simulink model "JCBL_Buck_Verify"  (R2024b)
settings: Solver=VariableStepAuto  StartTime=0.0  StopTime=0.5  RelTol=1e-3
undefined symbols (not defined in the file): C, L, RC, RL
libraries: spsCurrentMeasurementLib x9, spsMeanLib x6, spsVoltageMeasurementLib x6, spsSeriesRLCBranchLib x5, spsMosfetLib x4, spsOnDelayLib x4, slpidlib x3, simulink x3, eePowerMeasurement x2, spsRMSLib x2, spsControlledVoltageSourceLib x1, spsDCVoltageSourceLib x1
settings Model: Creator=admin  LastModifiedBy=admin
settings SolverCC: ZeroCrossAlgorithm=Adaptive  AlgebraicLoopSolver=TrustRegion
settings DebuggingCC: UnconnectedInputMsg=warning  UnconnectedOutputMsg=warning  UnconnectedLineMsg=warning
settings ModelReferenceCC: EnableRefExpFcnMdlSchedulingChecks=on
settings RTWCC: GPUComputeCapability=3.5  DLArmComputeVersion=19.05

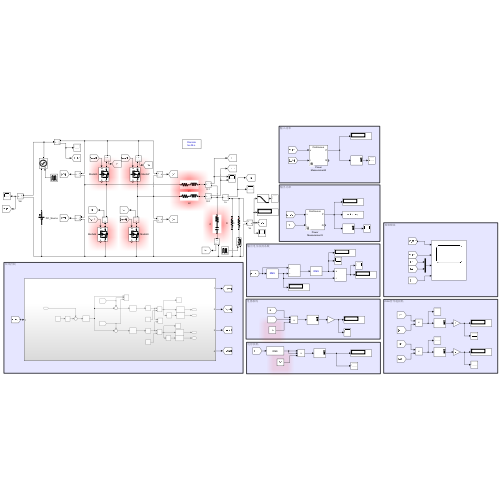
[thumbnail: Simulink's stored preview of the top-level diagram]
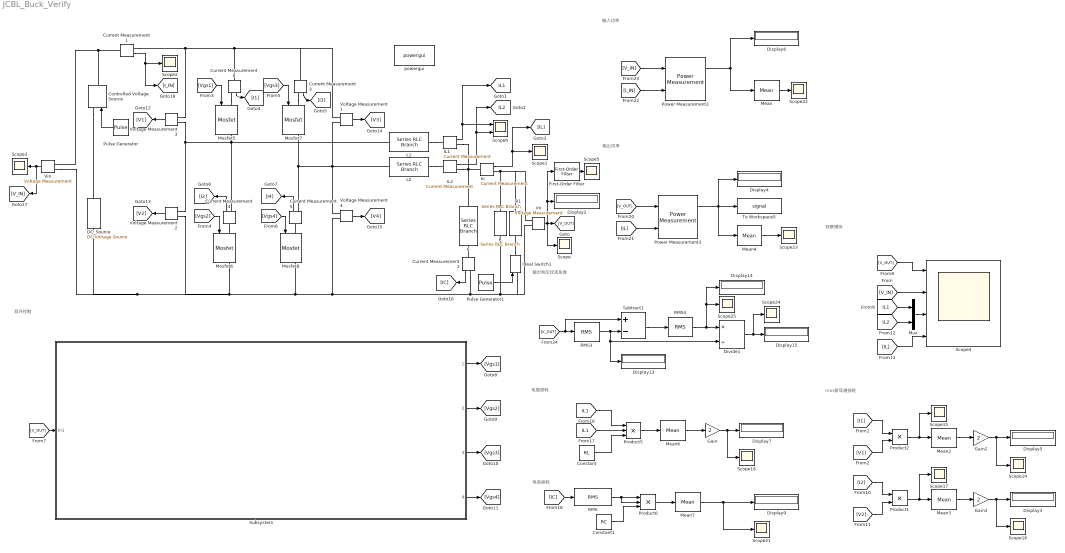
== system JCBL_Buck_Verify ==
  note: mos管导通损耗
  note: 电容损耗
  note: 电感损耗
  note: 输入功率
  note: 输出电压纹波系数
  note: 双环控制
  note: 输出功率
  note: 观察模块
  C : spsSeriesRLCBranchLib/Series RLC Branch  LConnTagsString=__new0  RConnTagsString=__new0  BranchType=RC  Resistance=RC  Inductance=1e-3  SetiL0=off  InitialCurrent=0  Capacitance=C  Setx0=off  InitialVoltage=0  Measurements=None
  Constant : Constant  Value=RL
  Constant1 : Constant  Value=RC
  Controlled Voltage Source : spsControlledVoltageSourceLib/Controlled Voltage Source  Initialize=on  Source_Type=AC  Amplitude=0  Phase=0  Frequency=0  Measurements=None
  Current Measurement{1..6} (6 alike) : spsCurrentMeasurementLib/Current Measurement  PhasorSimulation=off  OutputType=Complex  PSBequivalent=0
  DC_Source : spsDCVoltageSourceLib/DC Voltage Source  Amplitude=48  Measurements=None
  Display{2..7,9,13..15} (10 alike) : Display
  Divide1 : Product  Inputs=*/
  First-Order Filter : spsFirstOrderFilterLib/First-Order Filter  FilterType=Lowpass  Tc=1.26e-5  Ts=0  Initialize=off  Vac_Init=[0, 0, 60]  Vdc_Init=0  PlotResponse=off  FreqRange="[0,  200,  1]"
  Gain : Gain  Gain=2
  Gain2 : Gain  Gain=2
  Gain3 : Gain  Gain=2
  IL1 : spsCurrentMeasurementLib/Current Measurement  PhasorSimulation=off  OutputType=Complex  PSBequivalent=0
  IL2 : spsCurrentMeasurementLib/Current Measurement  PhasorSimulation=off  OutputType=Complex  PSBequivalent=0
  Ideal Switch1 : spsIdealSwitchLib/Ideal Switch  Ron=0.001  Lon=0  IC=0  Rs=1e5  Cs=inf  Measurements=off
  Io : spsCurrentMeasurementLib/Current Measurement  PhasorSimulation=off  OutputType=Complex  PSBequivalent=0
  L1 : spsSeriesRLCBranchLib/Series RLC Branch  LConnTagsString=__new0  RConnTagsString=__new0  BranchType=RL  Resistance=RL  Inductance=L  SetiL0=off  InitialCurrent=0  Capacitance=1e-6  Setx0=off  InitialVoltage=0  Measurements=None
  L2 : spsSeriesRLCBranchLib/Series RLC Branch  LConnTagsString=__new0  RConnTagsString=__new0  BranchType=RL  Resistance=RL  Inductance=L  SetiL0=off  InitialCurrent=0  Capacitance=1e-6  Setx0=off  InitialVoltage=0  Measurements=None
  Mean{,2..4,6..7} (6 alike) : spsMeanLib/Mean  Freq=500000  Vinit=0  Ts=0
  Mosfet{5..8} (4 alike) : spsMosfetLib/Mosfet  Ron=Ron  Lon=0  Rd=0.0001  Vfd=0  IC=0  Rs=1e5  Cs=inf  Measurements=on
  Mux : Mux  Inputs=2
  Power Measurement2 : eePowerMeasurement/Power Measurement  LabelModeActiveChoice=Continuous  F=60  K=[0]  Ts=0
  Power Measurement3 : eePowerMeasurement/Power Measurement  LabelModeActiveChoice=Continuous  F=60  K=[0]  Ts=0
  Product1 : Product
  Product2 : Product
  Product5 : Product  Inputs=3
  Product6 : Product  Inputs=3
  Pulse Generator : DiscretePulseGenerator  PulseType=Time based  Amplitude=4  Period=1  PulseWidth=15  PhaseDelay=0.25
  Pulse Generator1 : DiscretePulseGenerator  PulseType=Time based  Amplitude=4  Period=0.18  PulseWidth=1/3*100  PhaseDelay=0.16
  R : spsSeriesRLCBranchLib/Series RLC Branch  LConnTagsString=__new0  RConnTagsString=__new0  BranchType=R  Resistance=0.14  Inductance=1e-3  SetiL0=off  InitialCurrent=0  Capacitance=1e-6  Setx0=off  InitialVoltage=0  Measurements=None
  R1 : spsSeriesRLCBranchLib/Series RLC Branch  LConnTagsString=__new0  RConnTagsString=__new0  BranchType=R  Resistance=0.14  Inductance=1e-3  SetiL0=off  InitialCurrent=0  Capacitance=1e-6  Setx0=off  InitialVoltage=0  Measurements=None
  RMS : dspstat3/RMS  run=off  directionMode=Each column  dimension=1  InputProcessing=Columns as channels (frame based)  reset_popup=None
  RMS3 : spsRMSLib/RMS  TrueRMS=on  Freq=60  RMSInit=0  Ts=0
  RMS4 : spsRMSLib/RMS  TrueRMS=on  Freq=60  RMSInit=0  Ts=0
  Scope{,1..3,5,14..18,21..25} (15 alike) : Scope
  Scope4 : Scope  NumInputPorts=4
  Scope6 : Scope  NumInputPorts=2
  Subsystem : Subsystem
  Subtract1 : Sum  Inputs=+-
  To Workspace5 : ToWorkspace  VariableName=signal  SampleTime=0.1
  Vin : spsVoltageMeasurementLib/Voltage Measurement  PhasorSimulation=off  OutputType=Complex  PSBequivalent=0
  Vo : spsVoltageMeasurementLib/Voltage Measurement  PhasorSimulation=off  OutputType=Complex  PSBequivalent=0
  Voltage Measurement{1..4} (4 alike) : spsVoltageMeasurementLib/Voltage Measurement  PhasorSimulation=off  OutputType=Complex  PSBequivalent=0
  powergui : spspowerguiLib/powergui  Priority=1  SimulationMode=Discrete  SampleTime=5e-8  frequency=60  Iterations=50  frequencyindice=0  Pbase=100e6  ErrMax=1e-4  UnitsV=kV  UnitsW=MW  buscounter=0  FunctionMessages=off  echomessages=off  EnableUseOfTLC=off  CurrentSourceSwitches=off  DisableSnubberDevices=off  DisableRonSwitches=off  DisableVfSwitches=off  DisplayEquations=off  AutomaticDiscreteSolvers=off  SolverType=Tustin/Backward Euler (TBE)  Interpol=off  ExternalGateDelay=off  methode=off  Ts=100  x0status=blocks  SPID=on  SwTol=0  HookPort=off  NonlinearTolerance=1e-4  nMaxIteration=100  ContinueOnMaxIteration=off  RestoreLinks=warning  ResistiveCurrentMeasurement=off  Frange=[0:2:500]  Ylog=off  Xlog=on  ShowGrid=off  save=off  variable=ZData  structure=0  ZoomFFT=off  StartTime=0.0  cycles=1  DisplayStyle=1  fundamental=60  FreqAxis=off  MaxFrequency=1000  frequencyindicesteady=1  RmsSteady=1  display=off
  tag scope: IL1=global, IL2=global
  wires:
  Pulse Generator/1 -> Controlled Voltage Source/1
  Pulse Generator1/1 -> Ideal Switch1/1
  Gain3/1 -> Display3/1, Scope16/1
  Mean3/1 -> Gain3/1
  Gain2/1 -> Display5/1, Scope14/1
  Mean2/1 -> Gain2/1
  [I2] -> Product1/1
  [V2] -> Product1/2
  Product1/1 -> Mean3/1, Scope17/1
  Product2/1 -> Scope15/1, Mean2/1
  [V1] -> Product2/2
  [I1] -> Product2/1
  RMS/1 -> Product6/1, Product6/2
  Mean7/1 -> Display9/1, Scope21/1
  Product6/1 -> Mean7/1
  Constant1/1 -> Product6/3
  [IC] -> RMS/1
  Gain/1 -> Display7/1, Scope18/1
  Mean6/1 -> Gain/1
  Product5/1 -> Mean6/1
  Constant/1 -> Product5/3
  [IL1] -> Product5/2
  [IL1] -> Product5/1
  [V_IN] -> Power Measurement2/1
  [I_IN] -> Power Measurement2/2
  [IL] -> Power Measurement3/2
  [V_OUT] -> Power Measurement3/1
  Mean4/1 -> Scope23/1
  Power Measurement3/1 -> To Workspace5/1, Display4/1, Mean4/1
  Power Measurement2/1 -> Mean/1, Display6/1
  Mean/1 -> Scope22/1
  [V_OUT] -> Subtract1/1, RMS3/1
  RMS3/1 -> Subtract1/2, Divide1/2, Display13/1
  Subtract1/1 -> RMS4/1
  RMS4/1 -> Divide1/1, Display14/1, Scope25/1
  Divide1/1 -> Scope24/1, Display15/1
  [V_OUT] -> Subsystem/1(In1)
  Subsystem/4(4) -> [Vgs4]
  Subsystem/1(1) -> [Vgs1]
  Subsystem/2(2) -> [Vgs2]
  Subsystem/3(3) -> [Vgs3]
  [Vgs1] -> Mosfet5/1
  [Vgs3] -> Mosfet7/1
  Current Measurement5/1 -> [I4]
  Current Measurement6/1 -> [I1]
  Voltage Measurement4/1 -> [V4]
  Voltage Measurement3/1 -> [V1]
  [Vgs2] -> Mosfet6/1
  Voltage Measurement1/1 -> [V3]
  Voltage Measurement2/1 -> [V2]
  Current Measurement3/1 -> [I3]
  [Vgs4] -> Mosfet8/1
  Current Measurement4/1 -> [I2]
  Current Measurement2/1 -> [IC]
  Vin/1 -> [V_IN], Scope3/1
  Current Measurement1/1 -> Scope2/1, [I_IN]
  IL1/1 -> [IL1], Scope6/1
  IL2/1 -> [IL2], Scope6/2
  Io/1 -> [IL], Scope1/1
  Vo/1 -> Scope/1, First-Order Filter/1, Display2/1, [V_OUT]
  [IL1] -> Mux/1
  [IL2] -> Mux/2
  [V_OUT] -> Scope4/1
  [V_IN] -> Scope4/2
  Mux/1 -> Scope4/3
  [IL] -> Scope4/4
  First-Order Filter/1 -> Scope5/1
  connections:
  Current Measurement2/RConn1 -- Voltage Measurement4/LConn1 -- Voltage Measurement2/LConn1 -- Vin/LConn2 -- DC_Source/LConn1 -- Mosfet6/RConn1 -- Mosfet8/RConn1 -- Ideal Switch1/LConn1 -- Vo/LConn2 -- R/RConn1
  Controlled Voltage Source/RConn1 -- Vin/LConn1 -- Current Measurement1/LConn1
  C/LConn1 -- IL1/RConn1 -- Io/LConn1 -- IL2/RConn1
  Io/RConn1 -- R1/LConn1 -- Vo/LConn1 -- R/LConn1
  L2/RConn1 -- IL2/LConn1
  L1/RConn1 -- IL1/LConn1
  Current Measurement2/LConn1 -- C/RConn1
  Controlled Voltage Source/LConn1 -- DC_Source/RConn1
  Voltage Measurement3/LConn2 -- Voltage Measurement2/LConn2 -- L1/LConn1 -- Mosfet5/RConn1 -- Current Measurement4/RConn1
  Voltage Measurement1/LConn2 -- Voltage Measurement4/LConn2 -- Current Measurement5/RConn1 -- Mosfet7/RConn1 -- L2/LConn1
  Current Measurement4/LConn1 -- Mosfet6/LConn1
  Mosfet8/LConn1 -- Current Measurement5/LConn1
  Current Measurement3/RConn1 -- Mosfet7/LConn1
  Current Measurement6/RConn1 -- Mosfet5/LConn1
  Current Measurement1/RConn1 -- Voltage Measurement3/LConn1 -- Current Measurement3/LConn1 -- Voltage Measurement1/LConn1 -- Current Measurement6/LConn1
  Ideal Switch1/RConn1 -- R1/RConn1

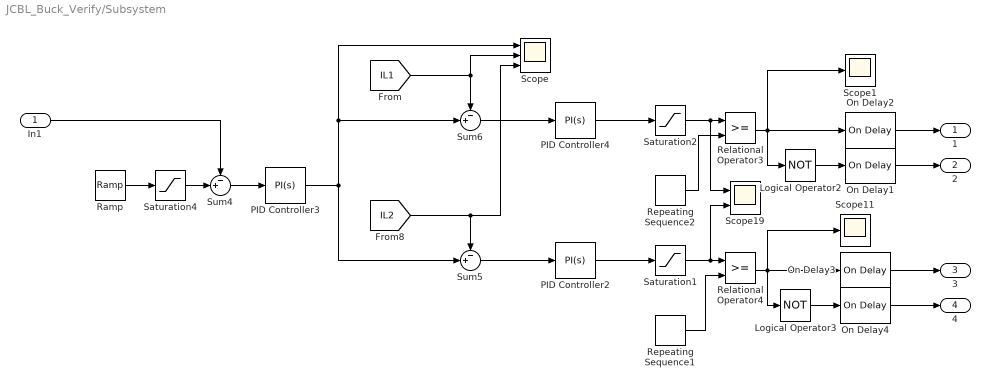
== system JCBL_Buck_Verify/Subsystem ==
  In1 : Inport
  Logical Operator2 : Logic  Operator=NOT  AllPortsSameDT=off  OutDataTypeStr=boolean
  Logical Operator3 : Logic  Operator=NOT  AllPortsSameDT=off  OutDataTypeStr=boolean
  On Delay{1..4} (4 alike) : spsOnDelayLib/On Delay  DelayType=On delay  delay=100e-9  ic=0  Ts=0
  PID Controller2 : slpidlib/PID Controller  Controller=PI  Form=Parallel  TimeDomain=Continuous-time  UseExternalTs=off  SampleTime=-1  IntegratorMethod=Forward Euler  FilterMethod=Forward Euler  ControllerParametersSource=internal  P=0.2  I=8  UseKiTs=off  D=0  UseExternalDerivativeSource=off  N=100  UseFilter=on  TunerSelectOption=Transfer Function Based (PID Tuner App)  InitialConditionSource=internal  InitialConditionForIntegrator=0  InitialConditionForFilter=0  DifferentiatorICPrevScaledInput=0  ExternalReset=none  TrackingMode=off  Kt=1  LimitOutput=on  SatLimitsSource=internal  UpperSaturationLimit=0.98  LowerSaturationLimit=0  LinearizeAsGain=on  AntiWindupMode=none  Kb=1  LimitIntegrator=off  UpperIntegratorSaturationLimit=0.95  LowerIntegratorSaturationLimit=0.05  POutMin=[]  POutMax=[]  IOutMin=[]  IOutMax=[]  DOutMin=[]  DOutMax=[]  NOutMin=[]  NOutMax=[]  SumOutMin=[]  SumOutMax=[]  SaturationOutMin=[]  SaturationOutMax=[]  PParamMin=[]  PParamMax=[]  IParamMin=[]  IParamMax=[]  DParamMin=[]  DParamMax=[]  NParamMin=[]  NParamMax=[]  KbParamMin=[]  KbParamMax=[]  KtParamMin=[]  KtParamMax=[]  KbOutMin=[]  KbOutMax=[]  KtOutMin=[]  KtOutMax=[]  IntegratorOutMin=[]  IntegratorOutMax=[]  FilterOutMin=[]  FilterOutMax=[]  SumI1OutMin=[]  SumI1OutMax=[]  SumI2OutMin=[]  SumI2OutMax=[]  SumI3OutMin=[]  SumI3OutMax=[]  SumI4OutMin=[]  SumI4OutMax=[]  SumDOutMin=[]  SumDOutMax=[]  DifferentiatorOutMin=[]  DifferentiatorOutMax=[]  FilterDiffOutCoefMin=[]  FilterDiffOutCoefMax=[]  ReciprocalOutMin=[]  ReciprocalOutMax=[]  SumDenOutMin=[]  SumDenOutMax=[]  SumNumOutMin=[]  SumNumOutMax=[]  DivideOutMin=[]  DivideOutMax=[]  UdiffTsProdOutMin=[]  UdiffTsProdOutMax=[]  NTsProdOutMin=[]  NTsProdOutMax=[]  UintegralTsProdOutMin=[]  UintegralTsProdOutMax=[]  UngainTsProdOutMin=[]  UngainTsProdOutMax=[]  ClampingZeroOutDataTypeStr=Inherit: Inherit via back propagation  ClampingZeroOutMin=[]  ClampingZeroOutMax=[]  FilterDenConstantOutDataTypeStr=Inherit: Inherit via back propagation  FilterDenConstantOutMin=[]  FilterDenConstantOutMax=[]  PCopyOutDataTypeStr=Inherit: Inherit via back propagation  PCopyOutMin=[]  PCopyOutMax=[]  NCopyOutDataTypeStr=Inherit: Inherit via back propagation  NCopyOutMin=[]  NCopyOutMax=[]  IntegratorContinuousStateAttributes=''  IntegratorStateMustResolveToSignalObject=off  IntegratorRTWStateStorageClass=Auto  FilterContinuousStateAttributes=''  FilterStateMustResolveToSignalObject=off  FilterRTWStateStorageClass=Auto  ParallelPVariant=InternalParameters  IdealPVariant=Disabled  IVariant=InternalParameters  DVariant=Disabled  IntegratorVariant=Continuous  SatVariant=Enabled  AWVariant=Passthrough  PCopyVariant=Disabled  TRVariant=Disabled  FdbkBlocksVariant=Forward  IdealPFdbkVariant=Disabled  SatFdbkVariant=Disabled  DerivativeFilterVariant=Disabled  NVariant=Disabled  NCopyVariant=Disabled_SignalSpec  FilterICVariant=Disabled  IntegratorICVariant=InternalICs  ExternalResetVariant=Disabled  TRSumVariant=Passthrough  SumFdbkVariant=Disabled  SumVariant=Sum_PI  TsampFilterVariant=InternalTs  TsampNgainVariant=Passthrough  TsampIntegralVariant=Disabled_SignalSpec  ExternalSaturationOutDataTypeStr=Inherit: Same as second input  DerivativeSourceVariant=Disabled  PreIntVariant=InternalPreInt
  PID Controller3 : slpidlib/PID Controller  Controller=PI  Form=Ideal  TimeDomain=Continuous-time  UseExternalTs=off  SampleTime=-1  IntegratorMethod=Forward Euler  FilterMethod=Forward Euler  ControllerParametersSource=internal  P=60  I=50  UseKiTs=off  D=0  UseExternalDerivativeSource=off  N=100  UseFilter=on  TunerSelectOption=Transfer Function Based (PID Tuner App)  InitialConditionSource=internal  InitialConditionForIntegrator=0  InitialConditionForFilter=0  DifferentiatorICPrevScaledInput=0  ExternalReset=none  TrackingMode=off  Kt=1  LimitOutput=on  SatLimitsSource=internal  UpperSaturationLimit=100  LowerSaturationLimit=0  LinearizeAsGain=on  AntiWindupMode=none  Kb=1  LimitIntegrator=off  UpperIntegratorSaturationLimit=4  LowerIntegratorSaturationLimit=0.05  POutMin=[]  POutMax=[]  IOutMin=[]  IOutMax=[]  DOutMin=[]  DOutMax=[]  NOutMin=[]  NOutMax=[]  SumOutMin=[]  SumOutMax=[]  SaturationOutMin=[]  SaturationOutMax=[]  PParamMin=[]  PParamMax=[]  IParamMin=[]  IParamMax=[]  DParamMin=[]  DParamMax=[]  NParamMin=[]  NParamMax=[]  KbParamMin=[]  KbParamMax=[]  KtParamMin=[]  KtParamMax=[]  KbOutMin=[]  KbOutMax=[]  KtOutMin=[]  KtOutMax=[]  IntegratorOutMin=[]  IntegratorOutMax=[]  FilterOutMin=[]  FilterOutMax=[]  SumI1OutMin=[]  SumI1OutMax=[]  SumI2OutMin=[]  SumI2OutMax=[]  SumI3OutMin=[]  SumI3OutMax=[]  SumI4OutMin=[]  SumI4OutMax=[]  SumDOutMin=[]  SumDOutMax=[]  DifferentiatorOutMin=[]  DifferentiatorOutMax=[]  FilterDiffOutCoefMin=[]  FilterDiffOutCoefMax=[]  ReciprocalOutMin=[]  ReciprocalOutMax=[]  SumDenOutMin=[]  SumDenOutMax=[]  SumNumOutMin=[]  SumNumOutMax=[]  DivideOutMin=[]  DivideOutMax=[]  UdiffTsProdOutMin=[]  UdiffTsProdOutMax=[]  NTsProdOutMin=[]  NTsProdOutMax=[]  UintegralTsProdOutMin=[]  UintegralTsProdOutMax=[]  UngainTsProdOutMin=[]  UngainTsProdOutMax=[]  ClampingZeroOutDataTypeStr=Inherit: Inherit via back propagation  ClampingZeroOutMin=[]  ClampingZeroOutMax=[]  FilterDenConstantOutDataTypeStr=Inherit: Inherit via back propagation  FilterDenConstantOutMin=[]  FilterDenConstantOutMax=[]  PCopyOutDataTypeStr=Inherit: Inherit via back propagation  PCopyOutMin=[]  PCopyOutMax=[]  NCopyOutDataTypeStr=Inherit: Inherit via back propagation  NCopyOutMin=[]  NCopyOutMax=[]  IntegratorContinuousStateAttributes=''  IntegratorStateMustResolveToSignalObject=off  IntegratorRTWStateStorageClass=Auto  FilterContinuousStateAttributes=''  FilterStateMustResolveToSignalObject=off  FilterRTWStateStorageClass=Auto  ParallelPVariant=Passthrough  IdealPVariant=InternalParameters  IVariant=InternalParameters  DVariant=Disabled  IntegratorVariant=Continuous  SatVariant=Enabled  AWVariant=Passthrough  PCopyVariant=Disabled  TRVariant=Disabled  FdbkBlocksVariant=Forward  IdealPFdbkVariant=Disabled  SatFdbkVariant=Disabled  DerivativeFilterVariant=Disabled  NVariant=Disabled  NCopyVariant=Disabled_SignalSpec  FilterICVariant=Disabled  IntegratorICVariant=InternalICs  ExternalResetVariant=Disabled  TRSumVariant=Passthrough  SumFdbkVariant=Disabled  SumVariant=Sum_PI  TsampFilterVariant=InternalTs  TsampNgainVariant=Passthrough  TsampIntegralVariant=Disabled_SignalSpec  ExternalSaturationOutDataTypeStr=Inherit: Same as second input  DerivativeSourceVariant=Disabled  PreIntVariant=InternalPreInt
  PID Controller4 : slpidlib/PID Controller  Controller=PI  Form=Parallel  TimeDomain=Continuous-time  UseExternalTs=off  SampleTime=-1  IntegratorMethod=Forward Euler  FilterMethod=Forward Euler  ControllerParametersSource=internal  P=0.2  I=8  UseKiTs=off  D=0  UseExternalDerivativeSource=off  N=100  UseFilter=on  TunerSelectOption=Transfer Function Based (PID Tuner App)  InitialConditionSource=internal  InitialConditionForIntegrator=0  InitialConditionForFilter=0  DifferentiatorICPrevScaledInput=0  ExternalReset=none  TrackingMode=off  Kt=1  LimitOutput=on  SatLimitsSource=internal  UpperSaturationLimit=0.98  LowerSaturationLimit=0  LinearizeAsGain=on  AntiWindupMode=none  Kb=1  LimitIntegrator=off  UpperIntegratorSaturationLimit=0.95  LowerIntegratorSaturationLimit=0.05  POutMin=[]  POutMax=[]  IOutMin=[]  IOutMax=[]  DOutMin=[]  DOutMax=[]  NOutMin=[]  NOutMax=[]  SumOutMin=[]  SumOutMax=[]  SaturationOutMin=[]  SaturationOutMax=[]  PParamMin=[]  PParamMax=[]  IParamMin=[]  IParamMax=[]  DParamMin=[]  DParamMax=[]  NParamMin=[]  NParamMax=[]  KbParamMin=[]  KbParamMax=[]  KtParamMin=[]  KtParamMax=[]  KbOutMin=[]  KbOutMax=[]  KtOutMin=[]  KtOutMax=[]  IntegratorOutMin=[]  IntegratorOutMax=[]  FilterOutMin=[]  FilterOutMax=[]  SumI1OutMin=[]  SumI1OutMax=[]  SumI2OutMin=[]  SumI2OutMax=[]  SumI3OutMin=[]  SumI3OutMax=[]  SumI4OutMin=[]  SumI4OutMax=[]  SumDOutMin=[]  SumDOutMax=[]  DifferentiatorOutMin=[]  DifferentiatorOutMax=[]  FilterDiffOutCoefMin=[]  FilterDiffOutCoefMax=[]  ReciprocalOutMin=[]  ReciprocalOutMax=[]  SumDenOutMin=[]  SumDenOutMax=[]  SumNumOutMin=[]  SumNumOutMax=[]  DivideOutMin=[]  DivideOutMax=[]  UdiffTsProdOutMin=[]  UdiffTsProdOutMax=[]  NTsProdOutMin=[]  NTsProdOutMax=[]  UintegralTsProdOutMin=[]  UintegralTsProdOutMax=[]  UngainTsProdOutMin=[]  UngainTsProdOutMax=[]  ClampingZeroOutDataTypeStr=Inherit: Inherit via back propagation  ClampingZeroOutMin=[]  ClampingZeroOutMax=[]  FilterDenConstantOutDataTypeStr=Inherit: Inherit via back propagation  FilterDenConstantOutMin=[]  FilterDenConstantOutMax=[]  PCopyOutDataTypeStr=Inherit: Inherit via back propagation  PCopyOutMin=[]  PCopyOutMax=[]  NCopyOutDataTypeStr=Inherit: Inherit via back propagation  NCopyOutMin=[]  NCopyOutMax=[]  IntegratorContinuousStateAttributes=''  IntegratorStateMustResolveToSignalObject=off  IntegratorRTWStateStorageClass=Auto  FilterContinuousStateAttributes=''  FilterStateMustResolveToSignalObject=off  FilterRTWStateStorageClass=Auto  ParallelPVariant=InternalParameters  IdealPVariant=Disabled  IVariant=InternalParameters  DVariant=Disabled  IntegratorVariant=Continuous  SatVariant=Enabled  AWVariant=Passthrough  PCopyVariant=Disabled  TRVariant=Disabled  FdbkBlocksVariant=Forward  IdealPFdbkVariant=Disabled  SatFdbkVariant=Disabled  DerivativeFilterVariant=Disabled  NVariant=Disabled  NCopyVariant=Disabled_SignalSpec  FilterICVariant=Disabled  IntegratorICVariant=InternalICs  ExternalResetVariant=Disabled  TRSumVariant=Passthrough  SumFdbkVariant=Disabled  SumVariant=Sum_PI  TsampFilterVariant=InternalTs  TsampNgainVariant=Passthrough  TsampIntegralVariant=Disabled_SignalSpec  ExternalSaturationOutDataTypeStr=Inherit: Same as second input  DerivativeSourceVariant=Disabled  PreIntVariant=InternalPreInt
  Ramp : simulink/Sources/Ramp  slope=240  start=0  InitialOutput=0
  Relational Operator3 : RelationalOperator  OutDataTypeStr=boolean  RndMeth=Simplest  InputSameDT=off
  Relational Operator4 : RelationalOperator  OutDataTypeStr=boolean  RndMeth=Simplest  InputSameDT=off
  Repeating Sequence1 : simulink/Sources/Repeating Sequence  rep_seq_t=[0 1/1000000 1/500000]  rep_seq_y=[1 0 1]
  Repeating Sequence2 : simulink/Sources/Repeating Sequence  rep_seq_t=[0 1/1000000 1/500000]  rep_seq_y=[0 1 0]
  Saturation1 : Saturate  UpperLimit=0.98  LowerLimit=0
  Saturation2 : Saturate  UpperLimit=0.98  LowerLimit=0
  Saturation4 : Saturate  UpperLimit=12  LowerLimit=0
  Scope : Scope  NumInputPorts=3
  Scope1 : Scope
  Scope11 : Scope
  Scope19 : Scope  NumInputPorts=2
  Sum4 : Sum  Inputs=-+|
  Sum5 : Sum  Inputs=-+|
  Sum6 : Sum  Inputs=-+|
  1 : Outport
  2 : Outport  Port=2
  3 : Outport  Port=3
  4 : Outport  Port=4
  wires:
  PID Controller2/1 -> Saturation1/1
  PID Controller4/1 -> Saturation2/1
  Repeating Sequence2/1 -> Relational Operator3/2
  Logical Operator2/1 -> On Delay1/1
  Saturation1/1 -> Scope19/2, Relational Operator4/1
  Sum4/1 -> PID Controller3/1
  Logical Operator3/1 -> On Delay4/1
  On Delay3/1 -> 3/1
  On Delay1/1 -> 2/1
  [IL2] -> Scope/3, Sum5/1
  Relational Operator3/1 -> Scope1/1, On Delay2/1, Logical Operator2/1
  Saturation2/1 -> Scope19/1, Relational Operator3/1
  Relational Operator4/1 -> On Delay3/1, Scope11/1, Logical Operator3/1
  On Delay2/1 -> 1/1
  [IL1] -> Sum6/1, Scope/2
  PID Controller3/1 -> Sum5/2, Scope/1, Sum6/2
  Ramp/1 -> Saturation4/1
  Sum5/1 -> PID Controller2/1
  In1/1 -> Sum4/1
  Sum6/1 -> PID Controller4/1
  Repeating Sequence1/1 -> Relational Operator4/2
  On Delay4/1 -> 4/1
  Saturation4/1 -> Sum4/2
